simulink model "Test1"  (R2016b)
settings: Solver=FixedStepAuto  StartTime=0.0  StopTime=inf  FixedStep=0.1  RelTol=1e-3  EnableMultiTasking=on
undefined symbols (not defined in the file or in its folder): pinNum
libraries: simulink_need_slupdate x11, EEE481Arduino x3, simulink x3, arduinolib x1
settings Model: ExtModeTrigDuration=2  Creator=rsjoshi1  LastModifiedBy=rsjoshi1
settings OptimizationCC: LifeSpan=1  MaxStackSize=64
settings DebuggingCC: SFUnexpectedBacktrackingDiag=warning  SFNoUnconditionalDefaultTransitionDiag=warning  SFExecutionAtInitializationDiag=none
settings HardwareCC: ProdBitPerPointer=32  ProdBitPerSizeT=32  ProdBitPerPtrDiffT=32  ProdLargestAtomicInteger=Long  ProdLargestAtomicFloat=Double  ProdWordSize=32  ProdHWDeviceType=ARM Compatible->ARM Cortex
settings RTWCC: SystemTargetFile=ert.tlc  HardwareBoard=Arduino Due  TLCOptions=-aInlineSetEventsForThisBaseRateFcn=TLC_FALSE -aSuppressMultiTaskScheduler=TLC_FALSE -aRateBasedStepFcn=1  TemplateMakefile=ert_default_tmf  Description=Embedded Coder  GenerateReport=on  Toolchain=Arduino ARM v1.6.7  BuildConfiguration=Faster Runs  IncludeHyperlinkInReport=on  LaunchReport=on  GenerateTraceInfo=on  GenerateTraceReport=on  GenerateTraceReportSl=on  GenerateTraceReportSf=on  GenerateTraceReportEml=on
settings CodeAppCC: ForceParamTrailComments=on  IgnoreCustomStorageClasses=off  OperatorAnnotations=on  SimulinkDataObjDesc=on  SFDataObjDesc=on  MATLABFcnDesc=on  InsertBlockDesc=on  MATLABSourceComments=on
settings ERTTargetCC: SupportContinuousTime=on  SupportVariableSizeSignals=on
settings ConfigComp: CovMetricSettings=dw  CovHtmlReporting=on  CovSaveCumulativeToWorkspaceVar=on  CovSaveSingleToWorkspaceVar=on  CovExternalEMLEnable=off

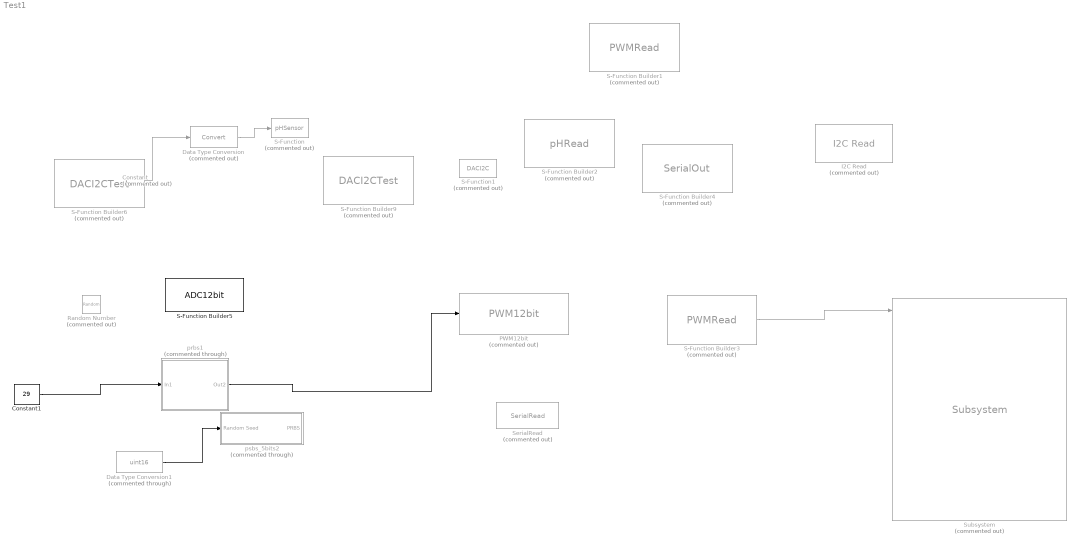
== system Test1 ==
  Constant : Constant  Commented=on
  Constant1 : Constant  Value=29  OutDataTypeStr=double  SampleTime=0.1
  Data Type Conversion : DataTypeConversion  Commented=on
  Data Type Conversion1 : DataTypeConversion  Commented=through  OutDataTypeStr=uint16
  I2C Read : arduinolib/I2C Read  Commented=on  SlaveAddress_=hex2dec( '61' )  RegisterAddressEnable=off  RegisterAddress_=hex2dec( '20' )  Datatype=uint8  ByteOrder=Big Endian  Datalength_=1  SampleTime_=1  blockPlatform=arduino
  PWM12bit : EEE481Arduino/PWM12bit  Commented=on  PwmPort=8  Tsa=0
  Random Number : RandomNumber  Commented=on  SampleTime=0.1
  S-Function : S-Function  Commented=on  FunctionName=pHSensor  Parameters=int8(1)  SFunctionModules=pHSensor_wrapper  SFunctionDeploymentMode=off  EnableBusSupport=off
  S-Function Builder1 : S-Function  Commented=on  InitFcn=try, set_param(gcb,'FunctionName','PWMRead'), end  FunctionName=PWMRead  SFunctionModules=PWMRead_wrapper  SFunctionDeploymentMode=off  EnableBusSupport=off  mask(S-Function Builder){}
      mask help: Simulink:masks:SFunctionBuilder_MD
      mask init:
      | val = [[.9  0.75 0.75 1 1 .9 .9 1]',[1 1 0.75 0.75 .9 .9 1 .9]'];try , sys = get_param(gcb,'SfunBuilderFcnName');if isempty(sys), sys = get_param(gcb,'FunctionName'); end,catch, sys = get_param(gcb,'FunctionName'); end
      settings: CopyFcn=set_param(gcbh,'LinkStatus','none')  PreSaveFcn=try, set_param(gcb,'FunctionName','PWMRead'), end  OpenFcn=sfunctionwizard(gcbh)
      mask Display: plot(val(:,1),val(:,2)),disp(sys), port_label('output',1,'PWMValue')
  S-Function Builder2 : S-Function  Commented=on  InitFcn=try, set_param(gcb,'FunctionName','pHRead'), end  FunctionName=pHRead  Parameters=int8(1)  SFunctionModules=pHRead_wrapper  SFunctionDeploymentMode=off  EnableBusSupport=off  mask(S-Function Builder){}
      mask help: Simulink:masks:SFunctionBuilder_MD
      mask init: same as Test1/S-Function Builder1
      settings: CopyFcn=set_param(gcbh,'LinkStatus','none')  PreSaveFcn=try, set_param(gcb,'FunctionName','pHRead'), end  OpenFcn=sfunctionwizard(gcbh)
      mask Display: plot(val(:,1),val(:,2)),disp(sys), port_label('input',1,'CommandNumber'), port_label('input',2,'TriggerCommand'), port_label('output',1,'pHValue')
  S-Function Builder3 : S-Function  Commented=on  InitFcn=try, set_param(gcb,'FunctionName','PWMRead'), end  FunctionName=PWMRead  SFunctionModules=PWMRead_wrapper  SFunctionDeploymentMode=off  EnableBusSupport=off  mask(S-Function Builder){}
      mask help: Simulink:masks:SFunctionBuilder_MD
      mask init: same as Test1/S-Function Builder1
      settings: CopyFcn=set_param(gcbh,'LinkStatus','none')  PreSaveFcn=try, set_param(gcb,'FunctionName','PWMRead'), end  OpenFcn=sfunctionwizard(gcbh)
      mask Display: plot(val(:,1),val(:,2)),disp(sys), port_label('output',1,'PWMValue')
  S-Function Builder4 : S-Function  Commented=on  InitFcn=try, set_param(gcb,'FunctionName','SerialOut'), end  FunctionName=SerialOut  Parameters=int8(0)  SFunctionModules=SerialOut_wrapper  SFunctionDeploymentMode=off  EnableBusSupport=off  mask(S-Function Builder){}
      mask help: Simulink:masks:SFunctionBuilder_MD
      mask init: same as Test1/S-Function Builder1
      settings: CopyFcn=set_param(gcbh,'LinkStatus','none')  PreSaveFcn=try, set_param(gcb,'FunctionName','SerialOut'), end  OpenFcn=sfunctionwizard(gcbh)
      mask Display: plot(val(:,1),val(:,2)),disp(sys), port_label('input',1,'input')
  S-Function Builder5 : S-Function  InitFcn=try, set_param(gcb,'FunctionName','ADC12bit'), end  FunctionName=ADC12bit  Parameters=int8(pinNum)  SFunctionModules=ADC12bit_wrapper  SFunctionDeploymentMode=off  EnableBusSupport=off  mask(S-Function Builder){}
      mask help: Simulink:masks:SFunctionBuilder_MD
      mask init: same as Test1/S-Function Builder1
      settings: CopyFcn=set_param(gcbh,'LinkStatus','none')  PreSaveFcn=try, set_param(gcb,'FunctionName','ADC12bit'), end  OpenFcn=sfunctionwizard(gcbh)
      mask Display:
      | plot(val(:,1),val(:,2))
      | disp(sys)
      | port_label('output',1,'output')
  S-Function Builder6 : S-Function  Commented=on  InitFcn=try, set_param(gcb,'FunctionName','DACI2CTest'), end  FunctionName=DACI2CTest  SFunctionModules=DACI2CTest_wrapper  SFunctionDeploymentMode=off  EnableBusSupport=off  mask(S-Function Builder){}
      mask help: Simulink:masks:SFunctionBuilder_MD
      mask init: same as Test1/S-Function Builder1
      settings: CopyFcn=set_param(gcbh,'LinkStatus','none')  PreSaveFcn=try, set_param(gcb,'FunctionName','DACI2CTest'), end  OpenFcn=sfunctionwizard(gcbh)
      mask Display:
      | plot(val(:,1),val(:,2))
      | disp(sys)
  S-Function Builder9 : S-Function  Commented=on  InitFcn=try, set_param(gcb,'FunctionName','DACI2CTest'), end  FunctionName=DACI2CTest  SFunctionModules=DACI2CTest_wrapper  SFunctionDeploymentMode=off  EnableBusSupport=off  mask(S-Function Builder){}
      mask help: Simulink:masks:SFunctionBuilder_MD
      mask init: same as Test1/S-Function Builder1
      settings: CopyFcn=set_param(gcbh,'LinkStatus','none')  PreSaveFcn=try, set_param(gcb,'FunctionName','DACI2CTest'), end  OpenFcn=sfunctionwizard(gcbh)
      mask Display:
      | plot(val(:,1),val(:,2))
      | disp(sys)
  S-Function1 : S-Function  Commented=on  FunctionName=DACI2C  SFunctionModules=DACI2C_wrapper  SFunctionDeploymentMode=off  EnableBusSupport=off
  SerialRead : EEE481Arduino/SerialRead  Commented=on  serialNum=2  Ts=1
  Subsystem : EEE481Arduino/Subsystem  Commented=on  Tsa=0.1  rate=1  per=0
  prbs1 : Subsystem  Commented=through
  psbs_5bits2 : Subsystem  Commented=through  mask(PRBS with 8 shift registers){T=1, Tsw=200, Lz=12000, Lv=100, Nc=1}
      mask prompts: T "Sample Time (s)"; Tsw "Time to switch (s)"; Lz "Leading Zeros (s)"; Lv "Switching Levels"; Nc "Number of Cycles"
      mask help:
      | Creates a PRBS signal using 6 shift registers.
      |     *Time to switch (Tsw) must be an integer multiple of Sample Time (T).
      |     *Leading zeros specify how long the PRBS will be zero, in seconds, before the levels begin shifting.
      |     *Level is the amplitude of the desired PRBS signal. Both + and - levels are equal
      |     *Number of cycles determines the number of full cycles generated. Each cycle is (2^6-1)*Tsw seconds long
  wires:
  Constant/1 -> Data Type Conversion/1
  Data Type Conversion/1 -> S-Function/1
  Data Type Conversion1/1 -> psbs_5bits2/1(Random Seed)
  prbs1/1(Out2) -> PWM12bit/1
  Constant1/1 -> prbs1/1(In1)
  S-Function Builder3/1 -> Subsystem/1

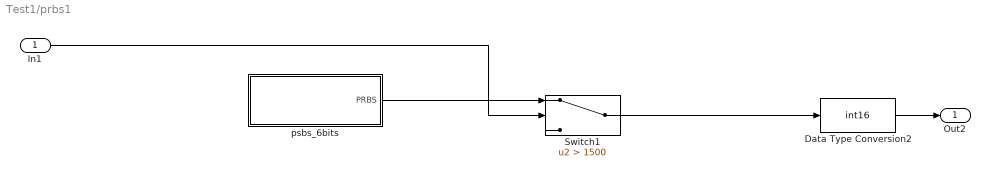
== system Test1/prbs1 ==
  In1 : Inport
  Data Type Conversion2 : DataTypeConversion  OutDataTypeStr=int16
  Switch1 : Switch  Criteria=u2 > Threshold  Threshold=1500
  psbs_6bits : Subsystem  mask(PRBS with 8 shift registers){T=0.1, Tsw=200, Lz=12000, Lv=60, Nc=100}
      mask prompts: T "Sample Time (s)"; Tsw "Time to switch (s)"; Lz "Leading Zeros (s)"; Lv "Switching Levels"; Nc "Number of Cycles"
      mask help:
      | Creates a PRBS signal using 6 shift registers.
      |     *Time to switch (Tsw) must be an integer multiple of Sample Time (T).
      |     *Leading zeros specify how long the PRBS will be zero, in seconds, before the levels begin shifting.
      |     *Level is the amplitude of the desired PRBS signal. Both + and - levels are equal
      |     *Number of cycles determines the number of full cycles generated. Each cycle is (2^6-1)*Tsw seconds long
  Out2 : Outport
  wires:
  Data Type Conversion2/1 -> Out2/1
  psbs_6bits/1(PRBS) -> Switch1/1
  Switch1/1 -> Data Type Conversion2/1
  In1/1 -> Switch1/2

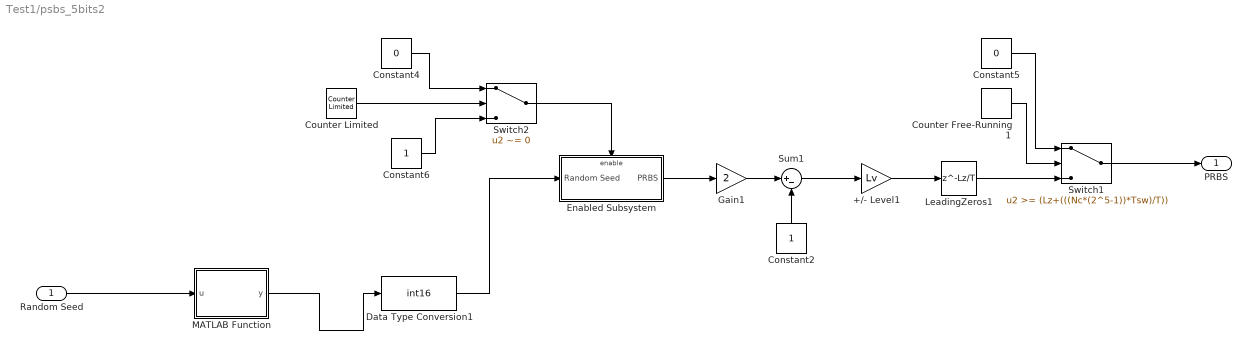
== system Test1/psbs_5bits2 ==
  Random Seed : Inport  OutDataTypeStr=uint16
  +/- Level1 : Gain  Gain=Lv  SampleTime=T
  Constant2 : Constant  SampleTime=T
  Constant4 : Constant  Value=0  SampleTime=T
  Constant5 : Constant  Value=0  SampleTime=T
  Constant6 : Constant  SampleTime=T
  Counter Free-Running1 : simulink/Sources/Counter Free-Running  NumBits=32  tsamp=T
  Counter Limited : simulink/Sources/Counter Limited  uplimit=Tsw/T-1  tsamp=T
  Data Type Conversion1 : DataTypeConversion  OutDataTypeStr=int16
  Enabled Subsystem : Subsystem  TreatAsAtomicUnit=on
  Gain1 : Gain  Gain=2  SampleTime=T
  LeadingZeros1 : Delay  DelayLength=Lz/T  InitialCondition=0  SampleTime=T
  MATLAB Function : MATLAB Function  TreatAsAtomicUnit=on
  Sum1 : Sum  Inputs=|+-  SampleTime=T
  Switch1 : Switch  Threshold=(Lz+(((Nc*(2^5-1))*Tsw)/T))  SampleTime=T
  Switch2 : Switch  Criteria=u2 ~= 0  Threshold=Tsw/T  SampleTime=T
  PRBS : Outport
  wires:
  Switch1/1 -> PRBS/1
  Random Seed/1 -> MATLAB Function/1(u)
  MATLAB Function/1(y) -> Data Type Conversion1/1
  LeadingZeros1/1 -> Switch1/3
  Constant5/1 -> Switch1/1
  +/- Level1/1 -> LeadingZeros1/1
  Counter Free-Running1/1 -> Switch1/2
  Constant2/1 -> Sum1/2
  Gain1/1 -> Sum1/1
  Sum1/1 -> +/- Level1/1
  Enabled Subsystem/1(PRBS) -> Gain1/1
  Data Type Conversion1/1 -> Enabled Subsystem/1(Random Seed)
  Constant6/1 -> Switch2/3
  Constant4/1 -> Switch2/1
  Switch2/1 -> Enabled Subsystem/Enable
  Counter Limited/1 -> Switch2/2

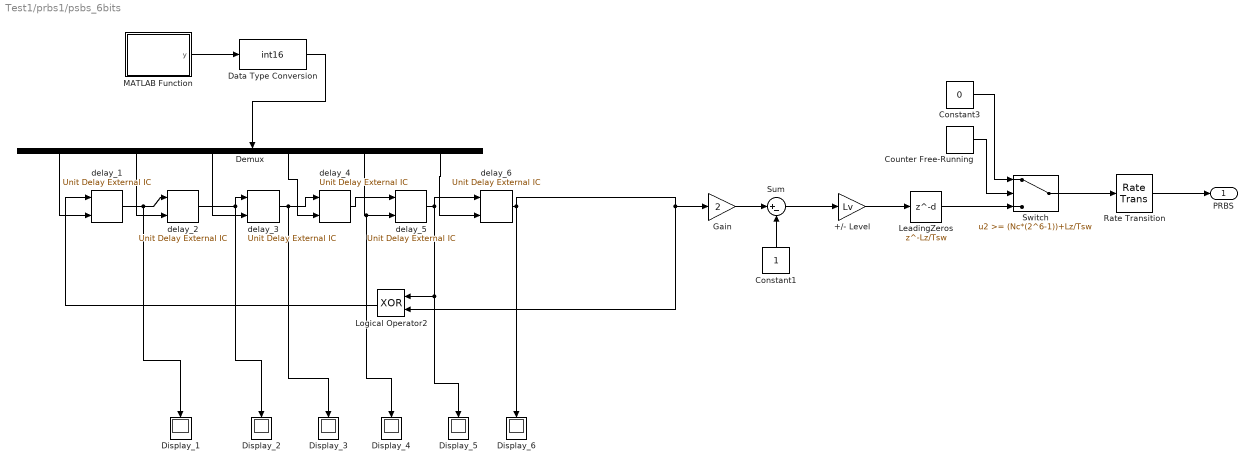
== system Test1/prbs1/psbs_6bits ==
  +/- Level : Gain  Gain=Lv  SampleTime=Tsw
  Constant1 : Constant  SampleTime=Tsw
  Constant3 : Constant  Value=0  SampleTime=Tsw
  Counter Free-Running : simulink/Sources/Counter Free-Running  NumBits=32  tsamp=Tsw
  Data Type Conversion : DataTypeConversion  OutDataTypeStr=int16  SampleTime=Tsw
  Demux : Demux  Outputs=6
  Display_{1..6} (6 alike) : Display
  Gain : Gain  Gain=2  SampleTime=Tsw
  LeadingZeros : Delay  DelayLength=Lz/Tsw  InitialCondition=0  SampleTime=Tsw
  Logical Operator2 : Logic  Operator=XOR  AllPortsSameDT=off  OutDataTypeStr=fixdt(1,16)  SampleTime=Tsw
  MATLAB Function : MATLAB Function  TreatAsAtomicUnit=on
  Rate Transition : RateTransition  OutPortSampleTime=T
  Sum : Sum  Inputs=|+-  SampleTime=Tsw
  Switch : Switch  Threshold=(Nc*(2^6-1))+Lz/Tsw  SampleTime=Tsw
  delay_{1..6} (6 alike) : simulink_need_slupdate/Unit Delay External IC  tsamp=Tsw
  PRBS : Outport
  wires:
  delay_5/1 -> Logical Operator2/1, Display_5/1, delay_6/1
  delay_2/1 -> Display_2/1, delay_3/1
  delay_3/1 -> Display_3/1, delay_4/1
  delay_4/1 -> delay_5/1
  delay_1/1 -> delay_2/1, Display_1/1
  delay_6/1 -> Logical Operator2/2, Gain/1, Display_6/1
  MATLAB Function/1(y) -> Data Type Conversion/1
  Demux/6 -> delay_6/2
  Demux/5 -> Display_4/1, delay_5/2
  Demux/4 -> delay_4/2
  Demux/3 -> delay_3/2
  Demux/2 -> delay_2/2
  Demux/1 -> delay_1/2
  Data Type Conversion/1 -> Demux/1
  Sum/1 -> +/- Level/1
  Gain/1 -> Sum/1
  Constant1/1 -> Sum/2
  Logical Operator2/1 -> delay_1/1
  Rate Transition/1 -> PRBS/1
  Counter Free-Running/1 -> Switch/2
  Switch/1 -> Rate Transition/1
  +/- Level/1 -> LeadingZeros/1
  Constant3/1 -> Switch/1
  LeadingZeros/1 -> Switch/3

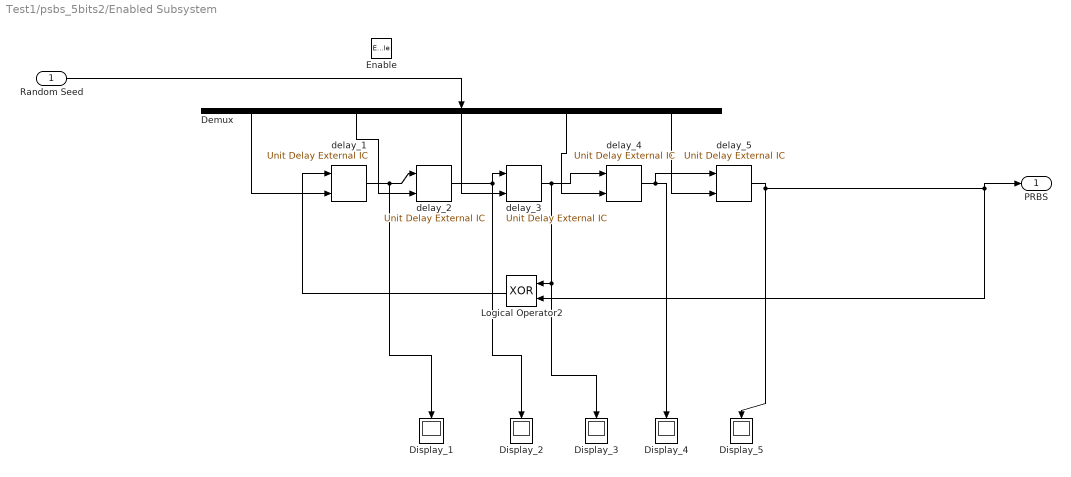
== system Test1/psbs_5bits2/Enabled Subsystem ==
  Random Seed : Inport  OutDataTypeStr=int16
  Enable : EnablePort
  Demux : Demux  Outputs=5
  Display_{1..5} (5 alike) : Display
  Logical Operator2 : Logic  Operator=XOR  AllPortsSameDT=off  OutDataTypeStr=fixdt(1,16)  SampleTime=T
  delay_{1..5} (5 alike) : simulink_need_slupdate/Unit Delay External IC  tsamp=T
  PRBS : Outport
  wires:
  delay_2/1 -> Display_2/1, delay_3/1
  delay_3/1 -> Display_3/1, Logical Operator2/1, delay_4/1
  delay_4/1 -> delay_5/1, Display_4/1
  delay_1/1 -> delay_2/1, Display_1/1
  Demux/5 -> delay_5/2
  Demux/4 -> delay_4/2
  Demux/3 -> delay_3/2
  Demux/2 -> delay_2/2
  Demux/1 -> delay_1/2
  Logical Operator2/1 -> delay_1/1
  delay_5/1 -> Display_5/1, PRBS/1, Logical Operator2/2
  Random Seed/1 -> Demux/1

== matlab function Test1/psbs_5bits2/MATLAB Function ==
  data: u input; y output
function y = fcn(u)
%#codegen
y = zeros(5,1);
% s = de2bi(u,16);
s = dec2bin(u,16);
y(1) = s(end-4)-48;
y(2) = s(end-3)-48;
y(3) = s(end-2)-48;
y(4) = s(end-1)-48;
y(5) = s(end)-48;

== matlab function Test1/prbs1/psbs_6bits/MATLAB Function ==
  data: y output
function y = fcn()
%#codegen
y = zeros(6,1);
% % s = de2bi(u,16);
% s = dec2bin(u,16);
s = ['1','1','0','1','0','0','1'];
y(1) = s(end-1)-48;
y(2) = s(end-2)-48;
y(3) = s(end-3)-48;
y(4) = s(end-4)-48;
y(5) = s(end-5)-48;
y(6) = s(end-6)-48;
